simulink model "MyDesignPTO"  (R2019b)
settings: Solver=ode4  StartTime=0  StopTime=200  FixedStep=sample_time  MaxStep=0.0025  RelTol=1e-3  EnableMultiTasking=on
values from neighbouring files (symbols this model uses):
  Am = 7.2    [value.m]
  Aw = 3.812*10^(-12)    (= 3.812e-12)    [value.m]
  depth = 5    [value.m]
  g = 9.81    [value.m]
  P_atmos = 101325    [value.m]
  rho = 1024    [value.m]
  valve_radius = 0.01    [value.m]
undefined symbols (not defined in the file or in its folder): sigbuilder_block
libraries: fl_lib x21, nesl_utility x12, sh_lib x8
settings Model: Creator=mlawson  LastModifiedBy=remil
settings SolverCC: ZeroCrossControl=DisableAll  AlgebraicLoopSolver=LineSearch  AutoInsertRateTranBlk=on
settings DataIOCC: SaveFormat=Array  SaveOutput=off  SaveTime=off  ReturnWorkspaceOutputs=off
settings OptimizationCC: LifeSpan=inf  SimCompilerOptimization=on
settings DebuggingCC: UnderspecifiedInitializationDetection=Classic  MergeDetectMultiDrivingBlocksExec=none  SolverPrmCheckMsg=warning  AllowSymbolicDim=off  StateNameClashWarn=warning  SFUnexpectedBacktrackingDiag=warning  SFNoUnconditionalDefaultTransitionDiag=warning  ArithmeticOperatorsInVariantConditions=warning
settings HardwareCC: ProdBitPerPointer=32  ProdBitPerSizeT=32  ProdBitPerPtrDiffT=32  ProdLargestAtomicFloat=None  ProdIntDivRoundTo=Undefined  ProdEndianess=Unspecified  ProdWordSize=32  ProdHWDeviceType=32-bit Generic
settings ModelReferenceCC: PropagateSignalLabelsOutOfModel=off
settings SFSimCC: SimUseLocalCustomCode=off  CustomCodeUndefinedFunction=UseInterfaceOnly
settings RTWCC: RTWUseLocalCustomCode=off
settings CodeAppCC: StateflowObjectComments=on
settings GRTTargetCC: TargetLangStandard=C89/C90 (ANSI)  GeneratePreprocessorConditionals=Disable all
settings ConfigComp: CovMetricSettings=dw  CovHtmlReporting=on  CovSaveCumulativeToWorkspaceVar=on  CovSaveSingleToWorkspaceVar=on  CovExternalEMLEnable=off  CovSFcnEnable=off
settings SimscapeCC: SimscapeNormalizeSystem=off  SimscapeLogType=all  SimscapeLogSimulationStatistics=on  SimscapeLogOpenViewer=on

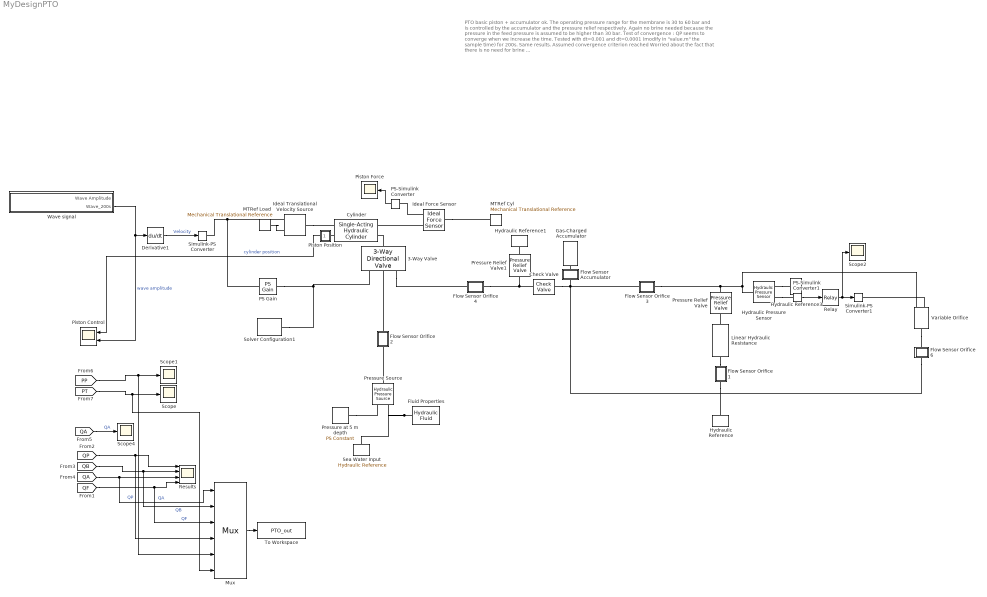
== system MyDesignPTO ==
  note: PTO basic piston + accumulator ok.
      | The operating pressure range for the membrane is 30 to 60 bar and is controlled by the accumulator and
      | the pressure relief respectively.
      | Again no brine needed because the pressure in the feed pressure is assumed to be higher than 30 bar.
      | Test of convergence : QP seems to converge when we increase the time.
      | Tested with dt=0.001 and dt=0.0001 (modify in "value.m" the sample time) for 200s. Same results. Assumed
      | convergence criterion reached
      |
      | Worried about the fact that there is no need for brine ...
  " Sea Water Input" : fl_lib/Hydraulic/Hydraulic Elements/Hydraulic Reference
      settings: SourceProductName=Simscape
  3-Way Valve : sh_lib/Valves/Directional Valves/3-Way Directional Valve  Tag=Factory Generic  area_spec=sh.valves.directional_valves.enum.area_spec.identical  x_0_P=0 m  x_0_T=0.08 m  mdl_type_identical=sh.valves.directional_valves.enum.mdl_type.linear  mdl_type_different=sh.valves.directional_valves.enum.mdl_type.linear  opening_max=2*valve_radius m  area_max=pi*(valve_radius)^2 m^2  opening_max_P_A=0.005 m  area_max_P_A=0.5e-4 m^2  opening_max_A_T=0.005 m  area_max_A_T=0.5e-4 m^2  opening_area_tab="[  -0.002 0 0.005 0.015 ] m"  area_tab="[  1e-12 4e-12 1e-05 1.02e-05 ] m^2"  opening_flow_rate_tab="[  -0.002 0 0.005 0.015 ] m"  pressure_tab="[  -5e+06 -2e+06 2e+06 5e+06 ] Pa"  flow_rate_tab="[  -1e-12 -6e-14 6e+12 1e+11 ; -8e-08 -4e-08 4e+06 8e+06 ; -0.0025 -0.00103 0.001 0.0024 ; -0.00258 -0.001032 0.00106 0.00247 ; ] m^3/s"  opening_area_tab_P_A=[-0.002, 0.0, 0.002, 0.005, 0.015] m  area_tab_P_A=[1.0e-9, 2.0352e-7, 4.0736e-5, 0.00011438, 0.00034356] m^2  opening_flow_rate_tab_P_A=[-0.002, 0.0, 0.002, 0.005, 0.015] m  pressure_tab_P_A=[-10000000.0, -5000000.0, -2000000.0, 2000000.0, 5000000.0, 10000000.0] Pa  flow_rate_tab_P_A=[-1.0e-7, -7.0711e-8, -4.4721e-8, 4.4721e-8, 7.0711e-8, 1.0e-7; -2.0352e-5, -1.4391e-5, -9.1017e-6, 9.1017e-6, 1.4391e-5, 2.0352e-5; -0.0040736, -0.0028805, -0.0018218, 0.0018218, 0.0028805, 0.0040736; -0.011438, -0.0080879, -0.0051152, 0.0051152, 0.0080879, 0.011438; -0.034356, -0.024293, -0.015364, 0.015364, 0.024293, 0.034356] m^3/s  opening_area_tab_A_T=[-0.002, 0.0, 0.002, 0.005, 0.015] m  area_tab_A_T=[1.0e-9, 2.0352e-7, 4.0736e-5, 0.00011438, 0.00034356] m^2  opening_flow_rate_tab_A_T=[-0.002, 0.0, 0.002, 0.005, 0.015] m  pressure_tab_A_T=[-10000000.0, -5000000.0, -2000000.0, 2000000.0, 5000000.0, 10000000.0] Pa  flow_rate_tab_A_T=[-1.0e-7, -7.0711e-8, -4.4721e-8, 4.4721e-8, 7.0711e-8, 1.0e-7; -2.0352e-5, -1.4391e-5, -9.1017e-6, 9.1017e-6, 1.4391e-5, 2.0352e-5; -0.0040736, -0.0028805, -0.0018218, 0.0018218, 0.0028805, 0.0040736; -0.011438, -0.0080879, -0.0051152, 0.0051152, 0.0080879, 0.011438; -0.034356, -0.024293, -0.015364, 0.015364, 0.024293, 0.034356] m^3/s  interp_method_identical=sh.valves.directional_valves.enum.interp_method.linear  interp_method_different=sh.valves.directional_valves.enum.interp_method.linear  extrap_method_identical=sh.valves.directional_valves.enum.extrap_method.linear  extrap_method_different=sh.valves.directional_valves.enum.extrap_method.linear  A_leak=1e-6 m^2  C_d=0.7  lam_spec=sh.valves.directional_valves.enum.lam_spec.pressure_ratio  B_lam=0.999  Re_cr=12
      settings: SourceProductName=Simscape Fluids  SourceProductBaseCode=SH  InternalSimscapePortConfiguration="{\"Bottom\":[],\"Left\":[{\"id\":\"A\",\"label\":\"A\",\"type\":\"foundation.hydraulic.hydraulic\"}],\"Right\":[{\"id\":\"S\",\"label\":\"S\",\"type\":\"input\"},{\"id\":\"P\",\"label\":\"P\",\"type\":\"foundation.hydraulic.hydraulic\"},{\"id\":\"T\",\"label\":\"T\",\"type\":\"foundation.hydraulic.hydraulic\"}],\"Top\":[]}"
  Check Valve : sh_lib/Valves/Directional Valves/Check Valve  Tag=Factory Generic  area_max=pi*(valve_radius)^2 m^2  pres_crack=30000 Pa  pres_max=120000 Pa  C_d=0.7  A_leak=1e-12 m^2  lam_spec=1  B_lam=0.999  Re_cr=12  dynamic=1  tau=0.1 s  area_init=1e-12 m^2
      settings: SourceProductName=Simscape Fluids  SourceProductBaseCode=SH  InternalSimscapePortConfiguration="{\"Bottom\":[],\"Left\":[{\"id\":\"A\",\"label\":\"A\",\"type\":\"foundation.hydraulic.hydraulic\"}],\"Right\":[{\"id\":\"B\",\"label\":\"B\",\"type\":\"foundation.hydraulic.hydraulic\"}],\"Top\":[]}"
  Cylinder : sh_lib/Hydraulic Cylinders/Single-Acting Hydraulic Cylinder  Tag=Factory Generic  area=top_piston_area m^2  stroke=piston_stroke m  init_pos=0 m  dead_vol=1e-06 m^3  init_pressure=0 Pa  k_sh=1.4  stiff=1e+07 N/m  D=250 N/(m/s)  hardstop_model=3  transition=0.1 mm  or=1
      settings: SourceProductName=Simscape Fluids  SourceProductBaseCode=SH  InternalSimscapePortConfiguration="{\"Bottom\":[],\"Left\":[{\"id\":\"C\",\"label\":\"C\",\"type\":\"foundation.mechanical.translational.translational\"},{\"id\":\"A\",\"label\":\"A\",\"type\":\"foundation.hydraulic.hydraulic\"}],\"Right\":[{\"id\":\"R\",\"label\":\"R\",\"type\":\"foundation.mechanical.translational.translational\"},{\"id\":\"P\",\"label\":\"P\",\"type\":\"output\"}],\"Top\":[]}"
  Derivative1 : Derivative
  Flow Sensor Accumulator : Subsystem
      mask Display: disp('QA')
  Flow Sensor Orifice 1 : Subsystem
      mask Display: disp('QP');
  Flow Sensor Orifice 2 : Subsystem
      mask Display: disp('PP');
  Flow Sensor Orifice 3 : Subsystem
      mask Display: disp('QF');
  Flow Sensor Orifice 4 : Subsystem
      mask Display: disp('PT');
  Flow Sensor Orifice 6 : Subsystem
      mask Display: disp('QB');
  Fluid Properties : sh_lib/Hydraulic Utilities/Hydraulic Fluid  Tag=Factory Generic  DataSource=1  SelFluid=1  SysTemp=40  TrapAir=0.002  ViscDerFactor=1  range_error=2
      settings: SourceProductName=Simscape Fluids
  Gas-Charged Accumulator : sh_lib/Accumulators/Gas-Charged Accumulator  capacity=2.5 gal  dead_volume=0.08 l  pr_preload=30e5 Pa  k_sh=1.4  stiff_coeff=1e12 Pa/m^3  penetr_coeff=1e10 s*Pa/m^6  flow_rate_specify=off  flow_rate_priority=High  flow_rate=0.005 m^3/s  flow_rate_nominal_specify=off  flow_rate_nominal_unit=m^3/s  flow_rate_nominal_value=1  liquid_volume_specify=on  liquid_volume_priority=High  liquid_volume=0 gal  liquid_volume_nominal_specify=off  liquid_volume_nominal_unit=m^3  liquid_volume_nominal_value=1  liquid_pressure_specify=off  liquid_pressure_priority=None  liquid_pressure=1.01325e+5 Pa  liquid_pressure_nominal_specify=off  liquid_pressure_nominal_unit=Pa  liquid_pressure_nominal_value=1
      settings: SourceProductName=Simscape Fluids  SourceProductBaseCode=SH  InternalSimscapePortConfiguration="{\"Bottom\":[],\"Left\":[],\"Right\":[{\"id\":\"A\",\"label\":\"A\",\"type\":\"foundation.hydraulic.hydraulic\"}],\"Top\":[]}"
  Hydraulic Pressure Sensor : fl_lib/Hydraulic/Hydraulic Sensors/Hydraulic Pressure Sensor
      settings: SourceProductName=Simscape
  Hydraulic Reference : fl_lib/Hydraulic/Hydraulic Elements/Hydraulic Reference
      settings: SourceProductName=Simscape
  Hydraulic Reference1 : fl_lib/Hydraulic/Hydraulic Elements/Hydraulic Reference
      settings: SourceProductName=Simscape
  Hydraulic Reference3 : fl_lib/Hydraulic/Hydraulic Elements/Hydraulic Reference
      settings: SourceProductName=Simscape
  Ideal Force Sensor : fl_lib/Mechanical/Mechanical Sensors/Ideal Force Sensor
  Ideal Translational Velocity Source : fl_lib/Mechanical/Mechanical Sources/Ideal Translational Velocity Source
  Linear Hydraulic Resistance : fl_lib/Hydraulic/Hydraulic Elements/Linear Hydraulic Resistance  resistance=1/(Am*Aw) Pa/(m^3/s)  q_specify=off  q_priority=None  q=0.001 m^3/s  q_nominal_specify=off  q_nominal_unit=m^3/s  q_nominal_value=1  p_specify=off  p_priority=None  p=0 Pa  p_nominal_specify=off  p_nominal_unit=Pa  p_nominal_value=1
      settings: SourceProductName=Simscape  SourceProductBaseCode=SS  InternalSimscapePortConfiguration="{\"Bottom\":[],\"Left\":[{\"id\":\"A\",\"label\":\"A\",\"type\":\"foundation.hydraulic.hydraulic\"}],\"Right\":[{\"id\":\"B\",\"label\":\"B\",\"type\":\"foundation.hydraulic.hydraulic\"}],\"Top\":[]}"
  MTRef Cyl : fl_lib/Mechanical/Translational Elements/Mechanical Translational Reference  Tag=Factory Generic
  MTRef Load : fl_lib/Mechanical/Translational Elements/Mechanical Translational Reference  Tag=Factory Generic
  Mux : Mux  Inputs=6
  PS Gain : fl_lib/Physical Signals/Functions/PS Gain  gain=1*valve_radius
  PS-Simulink Converter : nesl_utility/PS-Simulink Converter  PhysicalDomain=network_engine_domain  SubClassName=ps_output  LeftPortType=input  RightPortType=output  PseudoPeriodic=off  Frequencies=[]  Unit=inherit  AffineConversion=off
  PS-Simulink Converter1 : nesl_utility/PS-Simulink Converter  PhysicalDomain=network_engine_domain  SubClassName=ps_output  LeftPortType=input  RightPortType=output  PseudoPeriodic=off  Frequencies=[]  Unit=inherit  AffineConversion=off
  Piston Position : Subsystem
      mask Display: disp('P')
  Piston Control : Scope  NumInputPorts=2
  Piston Force : Scope
  Pressure Source : fl_lib/Hydraulic/Hydraulic Sources/Hydraulic Pressure Source  Tag=Factory Generic
      settings: SourceProductName=Simscape  SourceProductBaseCode=SS  InternalSimscapePortConfiguration="{\"Bottom\":[],\"Left\":[{\"id\":\"P\",\"label\":\"P\",\"type\":\"foundation.hydraulic.hydraulic\"}],\"Right\":[{\"id\":\"S\",\"label\":\"S\",\"type\":\"input\"},{\"id\":\"T\",\"label\":\"T\",\"type\":\"foundation.hydraulic.hydraulic\"}],\"Top\":[]}"
  Pressure Relief Valve : sh_lib/Valves/Pressure Control Valves/Pressure Relief Valve  valve_area_spec=1  p_diff_TLU=[30.15e5 : 15e3 : 31.35e5] Pa  area_TLU=[1 : 1 : 9] .* 1e-5 m^2  area_max=pi*(valve_radius)^2 m^2  pres_set=30e5 Pa  reg_range=5e5 Pa  C_d=0.7  A_leak=1e-12 m^2  lam_spec=1  B_lam=0.999  Re_cr=12  dynamic=0  tau=0.1 s  area_init=1e-12 m^2
      settings: SourceProductName=Simscape Fluids  SourceProductBaseCode=SH  InternalSimscapePortConfiguration="{\"Bottom\":[],\"Left\":[{\"id\":\"A\",\"label\":\"A\",\"type\":\"foundation.hydraulic.hydraulic\"}],\"Right\":[{\"id\":\"B\",\"label\":\"B\",\"type\":\"foundation.hydraulic.hydraulic\"}],\"Top\":[]}"
  Pressure Relief Valve1 : sh_lib/Valves/Pressure Control Valves/Pressure Relief Valve  valve_area_spec=1  p_diff_TLU=[30.15e5 : 15e3 : 31.35e5] Pa  area_TLU=[1 : 1 : 9] .* 1e-5 m^2  area_max=2*valve_radius m^2  pres_set=60*10^5 Pa  reg_range=5e5 Pa  C_d=0.7  A_leak=1e-12 m^2  lam_spec=1  B_lam=0.999  Re_cr=12  dynamic=0  tau=0.1 s  area_init=1e-12 m^2
      settings: SourceProductName=Simscape Fluids  SourceProductBaseCode=SH  InternalSimscapePortConfiguration="{\"Bottom\":[],\"Left\":[{\"id\":\"A\",\"label\":\"A\",\"type\":\"foundation.hydraulic.hydraulic\"}],\"Right\":[{\"id\":\"B\",\"label\":\"B\",\"type\":\"foundation.hydraulic.hydraulic\"}],\"Top\":[]}"
  Pressure at 5 m depth : fl_lib/Physical Signals/Sources/PS Constant  constant=P_atmos+rho*g*depth Pa
  Relay : Relay  OnSwitchValue=30*10^5  OffSwitchValue=0  OnOutputValue=0  OffOutputValue=2*valve_radius
  Results : Scope  NumInputPorts=4
  Scope{,1..2,4} (4 alike) : Scope
  Simulink-PS Converter : nesl_utility/Simulink-PS Converter  PhysicalDomain=network_engine_domain  SubClassName=ps_input  LeftPortType=input  RightPortType=output  PseudoPeriodic=off  Frequencies=[]  NoiseDistribution=none  NoiseParameters=[]  Unit=1  AffineConversion=off  FilteringAndDerivatives=filter  SimscapeFilterOrder=1  InputFilterTimeConstant=sample_time  UdotUserProvided=0
  Simulink-PS Converter1 : nesl_utility/Simulink-PS Converter  PhysicalDomain=network_engine_domain  SubClassName=ps_input  LeftPortType=input  RightPortType=output  PseudoPeriodic=off  Frequencies=[]  NoiseDistribution=none  NoiseParameters=[]  Unit=1  AffineConversion=off  FilteringAndDerivatives=filter  SimscapeFilterOrder=1  InputFilterTimeConstant=0.001  UdotUserProvided=0
  Solver Configuration1 : nesl_utility/Solver Configuration  PhysicalDomain=network_engine_domain  SubClassName=solver  LeftPortType=input  RightPortType=generic  Tones=[]  Harmonics=[]  SimulateNoise=off  Profile=off  UseLocalSampling=off  EnableSwitchedLinearOptims=on  FrequencyDomain=off  UseCCode=off  RelTol=0.001  AbsTol=1e-06  MinStep=1e-09  ToWorkspace=off  RevertToSquareIcSolve=off  NumHomotopyIterations=100  PhasorMode=off  PhasorModeNumHarmonics=1  DoDC=on  ResidualTolerance=1e-9  UseLocalSolver=on  LocalSolverChoice=NE_BACKWARD_EULER_ADVANCER  LocalSolverSampleTime=sample_time  DoFixedCost=on  MaxNonlinIter=3  MaxModeIter=2  LinearAlgebra=auto  EquationFormulation=NE_TIME_EF  DelaysMemoryBudget=1024  AutomaticFiltering=on  FilteringTimeConstant=sample_time  PartitionStorageMethod=AS_NEEDED  PartitionMemoryBudget=1024  PartitionMethod=FAST
  To Workspace : ToWorkspace  VariableName=PTO_out  SaveFormat=Structure With Time  SampleTime=-1
  Variable Orifice : sh_lib/Orifices/Variable Orifice  mdl_type=1  area_max=pi*(valve_radius)^2 m^2  opening_max=2*0.01 m  opening_tab=[-.002, 0, .002, .005, .015] m  area_tab=[1e-09, 2.0352e-07, 4.0736e-05, .00011438, .00034356] m^2  pressure_tab=[-10000000, -5000000, -2000000, 2000000, 5000000, 10000000] Pa  flow_rate_tab=[-1e-07, -7.0711e-08, -4.4721e-08, 4.4721e-08, 7.0711e-08, 1e-07; -2.0352e-05, -1.4391e-05, -9.1017e-06, 9.1017e-06, 1.4391e-05, 2.0352e-05; -.0040736, -.0028805, -.0018218, .0018218, .0028805, .0040736; -.011438, -.0080879, -.0051152, .0051152, .0080879, .011438; -.034356, -.024293, -.015364, .015364, .024293, .034356] m^3/s  interp_method=1  extrap_method=1  or=1  C_d=0.7  x_0=0 m  A_leak=1e-12 m^2  lam_spec=1  B_lam=0.999  Re_cr=12  flow_rate_specify=off  flow_rate_priority=High  flow_rate=0 m^3/s  flow_rate_nominal_specify=off  flow_rate_nominal_unit=m^3/s  flow_rate_nominal_value=1  pressure_drop_specify=off  pressure_drop_priority=None  pressure_drop=0 Pa  pressure_drop_nominal_specify=off  pressure_drop_nominal_unit=Pa  pressure_drop_nominal_value=1
      settings: SourceProductName=Simscape Fluids  SourceProductBaseCode=SH  InternalSimscapePortConfiguration="{\"Bottom\":[],\"Left\":[{\"id\":\"S\",\"label\":\"S\",\"type\":\"input\"},{\"id\":\"A\",\"label\":\"A\",\"type\":\"foundation.hydraulic.hydraulic\"}],\"Right\":[{\"id\":\"B\",\"label\":\"B\",\"type\":\"foundation.hydraulic.hydraulic\"}],\"Top\":[]}"
  Wave signal : Subsystem  Tag=STV Subsys  LoadFcn=sigbuilder_block('load');  StartFcn=sigbuilder_block('start');  StopFcn=sigbuilder_block('stop');  ClipboardFcn=sigbuilder_block('clipboard');  mask(Sigbuilder block){tuvar=[0:10]}
      mask help: Simulink:masks:SigbuilderBlock_MD
      mask init:
      | if ~strcmp(get_param(bdroot(gcbh),'SimulationStatus'),'stopped') tuvar = sigbuilder_block('maskInit'); end
      settings: CopyFcn=sigbuilder_block('copy');  DeleteFcn=sigbuilder_block('delete');  ModelCloseFcn=sigbuilder_block('modelClose');  PreSaveFcn=sigbuilder_block('preSave');  PauseFcn=sigbuilder_block('pause');  ContinueFcn=sigbuilder_block('continue');  NameChangeFcn=sigbuilder_block('namechange');  OpenFcn=sigbuilder_block('open',[437.6 199.2 550.4 400 ]);  CloseFcn=sigbuilder_block('close');
      mask Display: plot(0, 0, 100, 100,[2, 2, 32, 32, 2], [68, 8, 8, 68, 68],[32, 2], [38, 38], [32, 19, 2],[53, 60, 44], [32, 17, 17, 2],[16, 16, 31, 31]);txt = getActiveGroup(gcbh);text(2, 100, txt,'verticalAlignment', 'top');
  wires:
  Piston Position/1(Out1) -> Piston Control/1  "cylinder position"
  Wave signal/2(Wave_200s) -> Piston Control/2, Derivative1/1  "wave amplitude"
  PS-Simulink Converter/1 -> Piston Force/1
  [PT] -> Mux/6, Scope/1
  [PP] -> Mux/5, Scope1/1
  [QF] -> Mux/3, Results/4  "QF"
  [QB] -> Mux/2, Results/2  "QB"
  [QA] -> Scope4/1  "QA"
  [QP] -> Mux/4, Results/1  "QP"
  [QA] -> Mux/1, Results/3  "QA"
  Derivative1/1 -> Simulink-PS Converter/1  "Velocity"
  PS-Simulink Converter1/1 -> Relay/1
  Relay/1 -> Scope2/1, Simulink-PS Converter1/1
  Mux/1 -> To Workspace/1
  connections:
  Ideal Translational Velocity Source/LConn1 -- Cylinder/RConn1
  Fluid Properties/RConn1 -- " Sea Water Input"/LConn1 -- Pressure Source/RConn2
  Cylinder/RConn2 -- Piston Position/LConn1
  3-Way Valve/LConn1 -- Cylinder/LConn2
  Solver Configuration1/RConn1 -- 3-Way Valve/RConn1 -- PS Gain/RConn1
  Pressure at 5 m depth/RConn1 -- Pressure Source/RConn1
  MTRef Load/LConn1 -- Ideal Translational Velocity Source/RConn2
  Simulink-PS Converter/RConn1 -- PS Gain/LConn1 -- Ideal Translational Velocity Source/RConn1
  Ideal Force Sensor/LConn1 -- MTRef Cyl/LConn1
  Ideal Force Sensor/RConn1 -- Cylinder/LConn1
  Ideal Force Sensor/RConn2 -- PS-Simulink Converter/LConn1
  Check Valve/RConn1 -- Flow Sensor Orifice 3/LConn1 -- Flow Sensor Orifice 6/LConn1 -- Flow Sensor Accumulator/LConn1
  Linear Hydraulic Resistance/LConn1 -- Pressure Relief Valve/RConn1
  Linear Hydraulic Resistance/RConn1 -- Flow Sensor Orifice 1/LConn1
  Gas-Charged Accumulator/RConn1 -- Flow Sensor Accumulator/RConn1
  Flow Sensor Orifice 1/RConn1 -- Hydraulic Reference/LConn1
  Flow Sensor Orifice 3/RConn1 -- Hydraulic Pressure Sensor/LConn1 -- Variable Orifice/LConn2 -- Pressure Relief Valve/LConn1
  3-Way Valve/RConn3 -- Flow Sensor Orifice 4/LConn1
  Flow Sensor Orifice 4/RConn1 -- Pressure Relief Valve1/LConn1 -- Check Valve/LConn1
  Pressure Source/LConn1 -- Flow Sensor Orifice 2/LConn1
  Flow Sensor Orifice 2/RConn1 -- 3-Way Valve/RConn2
  Hydraulic Reference1/LConn1 -- Pressure Relief Valve1/RConn1
  Hydraulic Pressure Sensor/RConn1 -- Hydraulic Reference3/LConn1
  Hydraulic Pressure Sensor/RConn2 -- PS-Simulink Converter1/LConn1
  Variable Orifice/RConn1 -- Flow Sensor Orifice 6/RConn1
  Variable Orifice/LConn1 -- Simulink-PS Converter1/RConn1

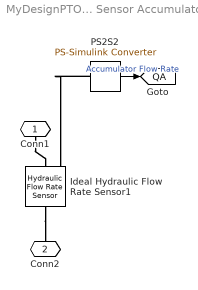
== system MyDesignPTO/Flow Sensor Accumulator ==
  Ideal Hydraulic Flow Rate Sensor1 : fl_lib/Hydraulic/Hydraulic Sensors/Hydraulic Flow Rate Sensor  Tag=Factory Generic
      settings: SourceProductName=Simscape
  PS2S2 : nesl_utility/PS-Simulink Converter  PhysicalDomain=network_engine_domain  SubClassName=ps_output  LeftPortType=input  RightPortType=output  PseudoPeriodic=off  Frequencies=[]  Unit=1  AffineConversion=off
  Conn1 : PMIOPort  Side=Right
  Conn2 : PMIOPort  Port=2  Side=Left
  tag scope: QA=global
  wires:
  PS2S2/1 -> [QA]  "Accumulator Flow Rate"
  connections:
  PS2S2/LConn1 -- Ideal Hydraulic Flow Rate Sensor1/RConn1
  Conn1/RConn1 -- Ideal Hydraulic Flow Rate Sensor1/RConn2
  Ideal Hydraulic Flow Rate Sensor1/LConn1 -- Conn2/RConn1

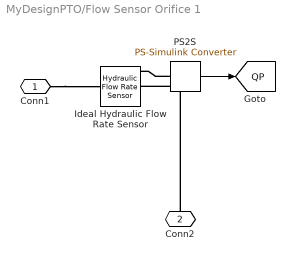
== system MyDesignPTO/Flow Sensor Orifice 1 ==
  Ideal Hydraulic Flow Rate Sensor : fl_lib/Hydraulic/Hydraulic Sensors/Hydraulic Flow Rate Sensor  Tag=Factory Generic
      settings: SourceProductName=Simscape
  PS2S : nesl_utility/PS-Simulink Converter  PhysicalDomain=network_engine_domain  SubClassName=ps_output  LeftPortType=input  RightPortType=output  PseudoPeriodic=off  Frequencies=[]  Unit=1  AffineConversion=off
  Conn1 : PMIOPort  Side=Left
  Conn2 : PMIOPort  Port=2  Side=Right
  tag scope: QP=global
  wires:
  PS2S/1 -> [QP]
  connections:
  PS2S/LConn1 -- Ideal Hydraulic Flow Rate Sensor/RConn1
  Conn2/RConn1 -- Ideal Hydraulic Flow Rate Sensor/RConn2
  Conn1/RConn1 -- Ideal Hydraulic Flow Rate Sensor/LConn1

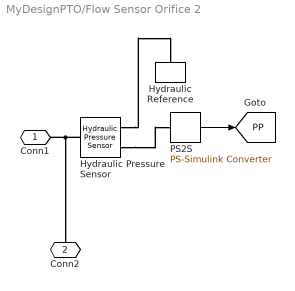
== system MyDesignPTO/Flow Sensor Orifice 2 ==
  Hydraulic Pressure Sensor : fl_lib/Hydraulic/Hydraulic Sensors/Hydraulic Pressure Sensor
      settings: SourceProductName=Simscape
  Hydraulic Reference : fl_lib/Hydraulic/Hydraulic Elements/Hydraulic Reference
      settings: SourceProductName=Simscape
  PS2S : nesl_utility/PS-Simulink Converter  PhysicalDomain=network_engine_domain  SubClassName=ps_output  LeftPortType=input  RightPortType=output  PseudoPeriodic=off  Frequencies=[]  Unit=1  AffineConversion=off
  Conn1 : PMIOPort  Side=Left
  Conn2 : PMIOPort  Port=2  Side=Right
  tag scope: PP=global
  wires:
  PS2S/1 -> [PP]
  connections:
  Conn1/RConn1 -- Hydraulic Pressure Sensor/LConn1 -- Conn2/RConn1
  Hydraulic Pressure Sensor/RConn2 -- PS2S/LConn1
  Hydraulic Pressure Sensor/RConn1 -- Hydraulic Reference/LConn1

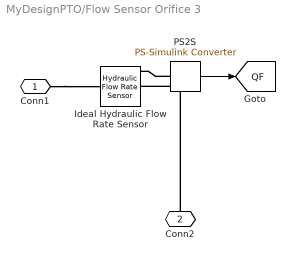
== system MyDesignPTO/Flow Sensor Orifice 3 ==
  Ideal Hydraulic Flow Rate Sensor : fl_lib/Hydraulic/Hydraulic Sensors/Hydraulic Flow Rate Sensor  Tag=Factory Generic
      settings: SourceProductName=Simscape
  PS2S : nesl_utility/PS-Simulink Converter  PhysicalDomain=network_engine_domain  SubClassName=ps_output  LeftPortType=input  RightPortType=output  PseudoPeriodic=off  Frequencies=[]  Unit=1  AffineConversion=off
  Conn1 : PMIOPort  Side=Left
  Conn2 : PMIOPort  Port=2  Side=Right
  tag scope: QF=global
  wires:
  PS2S/1 -> [QF]
  connections:
  PS2S/LConn1 -- Ideal Hydraulic Flow Rate Sensor/RConn1
  Conn2/RConn1 -- Ideal Hydraulic Flow Rate Sensor/RConn2
  Conn1/RConn1 -- Ideal Hydraulic Flow Rate Sensor/LConn1

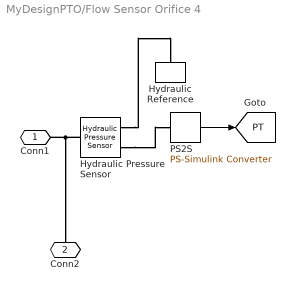
== system MyDesignPTO/Flow Sensor Orifice 4 ==
  Hydraulic Pressure Sensor : fl_lib/Hydraulic/Hydraulic Sensors/Hydraulic Pressure Sensor
      settings: SourceProductName=Simscape
  Hydraulic Reference : fl_lib/Hydraulic/Hydraulic Elements/Hydraulic Reference
      settings: SourceProductName=Simscape
  PS2S : nesl_utility/PS-Simulink Converter  PhysicalDomain=network_engine_domain  SubClassName=ps_output  LeftPortType=input  RightPortType=output  PseudoPeriodic=off  Frequencies=[]  Unit=1  AffineConversion=off
  Conn1 : PMIOPort  Side=Left
  Conn2 : PMIOPort  Port=2  Side=Right
  tag scope: PT=global
  wires:
  PS2S/1 -> [PT]
  connections:
  Hydraulic Pressure Sensor/LConn1 -- Conn2/RConn1 -- Conn1/RConn1
  Hydraulic Pressure Sensor/RConn2 -- PS2S/LConn1
  Hydraulic Pressure Sensor/RConn1 -- Hydraulic Reference/LConn1

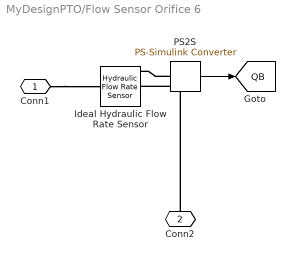
== system MyDesignPTO/Flow Sensor Orifice 6 ==
  Ideal Hydraulic Flow Rate Sensor : fl_lib/Hydraulic/Hydraulic Sensors/Hydraulic Flow Rate Sensor  Tag=Factory Generic
      settings: SourceProductName=Simscape
  PS2S : nesl_utility/PS-Simulink Converter  PhysicalDomain=network_engine_domain  SubClassName=ps_output  LeftPortType=input  RightPortType=output  PseudoPeriodic=off  Frequencies=[]  Unit=1  AffineConversion=off
  Conn1 : PMIOPort  Side=Left
  Conn2 : PMIOPort  Port=2  Side=Right
  tag scope: QB=global
  wires:
  PS2S/1 -> [QB]
  connections:
  PS2S/LConn1 -- Ideal Hydraulic Flow Rate Sensor/RConn1
  Conn2/RConn1 -- Ideal Hydraulic Flow Rate Sensor/RConn2
  Conn1/RConn1 -- Ideal Hydraulic Flow Rate Sensor/LConn1

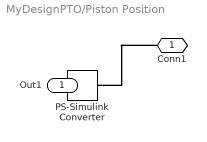
== system MyDesignPTO/Piston Position ==
  PS-Simulink Converter : nesl_utility/PS-Simulink Converter  PhysicalDomain=network_engine_domain  SubClassName=ps_output  LeftPortType=input  RightPortType=output  PseudoPeriodic=off  Frequencies=[]  Unit=1  AffineConversion=off
  Conn1 : PMIOPort  Side=Left
  Out1 : Outport  VectorParamsAs1DForOutWhenUnconnected=off
  wires:
  PS-Simulink Converter/1 -> Out1/1
  connections:
  Conn1/RConn1 -- PS-Simulink Converter/LConn1

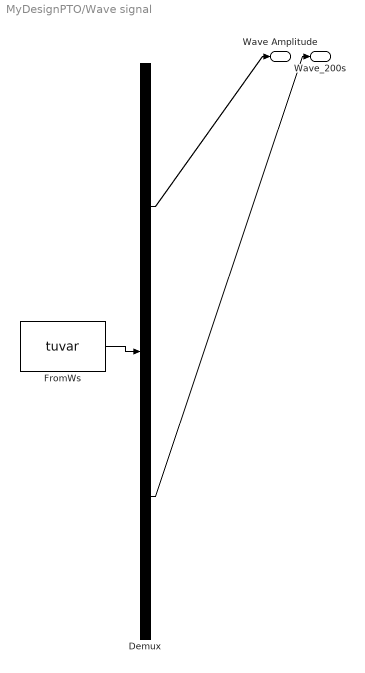
== system MyDesignPTO/Wave signal ==
  Demux : Demux  Tag=STV Demux  Outputs=2
  FromWs : FromWorkspace  Tag=STV FromWs  VariableName=tuvar  SampleTime=0
      SigBuilderData=|
      | common.afterFinalStr = 'Extrapolate'
      | common.sampleTime = 0
      | dataSet.timeRange = [0 200]
      | dataSet.name = 'Group 1'
      | sbobj.Groups.Name = 'Group 1'
      | sbobj.Groups.Signals(1).Name = 'Wave Amplitude'
      | sbobj.Groups.Signals(1).XData = [0 0.0140280561122 0.0280561122244 0.0420841683367 0.0561122244489 0.0701402805611 0.0841683366733 0.0981963927856 0.112224448898 0.12625250501 0.140280561122 0.154308617234 ... (3567 elements, 1x3567)]
      | sbobj.Groups.Signals(1).YData = [0 0.0125912209985 0.0251804457201 0.0377656782048 0.050344923125 0.0629161861029 0.0754774740258 0.0880267953628 0.10056216048 0.113081581956 0.125583074899 0.138064657256 ... (3567 elements, 1x3567)]
      | sbobj.Groups.Signals(2).Name = 'Wave_200s'
      | sbobj.Groups.Signals(2).XData = [0 0.0140280561122 0.0280561122244 0.0420841683367 0.0561122244489 0.0701402805611 0.0841683366733 0.0981963927856 0.112224448898 0.12625250501 0.140280561122 0.154308617234 ... (14259 elements, 1x14259)]
      | sbobj.Groups.Signals(2).YData = [0 0.0125912209985 0.0251804457201 0.0377656782048 0.050344923125 0.0629161861029 0.0754774740258 0.0880267953628 0.10056216048 0.113081581956 0.125583074899 0.138064657256 ... (14259 elements, 1x14259)]
      | sbobj.Groups.TimeRange = [0 200]
  Wave Amplitude : Outport  Tag=STV Outport
  Wave_200s : Outport  Tag=STV Outport  Port=2
  wires:
  FromWs/1 -> Demux/1
  Demux/1 -> Wave Amplitude/1
  Demux/2 -> Wave_200s/1
